simulink model "PLANT_LAB4"  (R2025b)
settings: Solver=VariableStepAuto  StartTime=0.0  StopTime=10.0  RelTol=1e-3
values from neighbouring files (symbols this model uses):
  C12 = -(batt.m*46.05+2*mot.rot.m*-7)*r    [CM_LAB4.m]
  F = [F11 F12; F12 F22]    [CM_LAB4.m]
  G2 = -(batt.m*46.05+2*mot.rot.m*-7)*g    [CM_LAB4.m]
  M11 = 2*wheel.Iyy + 2*gbox.N^2*mot.rot.Iyy+(batt.m+2*wheel.m+2*mot.m)*r^2    [CM_LAB4.m]
  M21_1 = 2*gbox.N*(1-gbox.N)*mot.rot.Iyy    [CM_LAB4.m]
  M21_2 = (batt.m*46.05+2*mot.rot.m*-7)*r    [CM_LAB4.m]
  M22 = batt.Iyy+2*(1-gbox.N)^2*mot.rot.Iyy+batt.m*46.05^2+2*mot.rot.m*49    [CM_LAB4.m]
  r = sqrt((2.20*2)/1.06)    [CM_LAB4.m]
undefined symbols (not defined in the file or in its folder): drv, g, gbox, mot, ms22g, sens, Ts
settings Model: Creator=Gioele  LastModifiedBy=Gioele

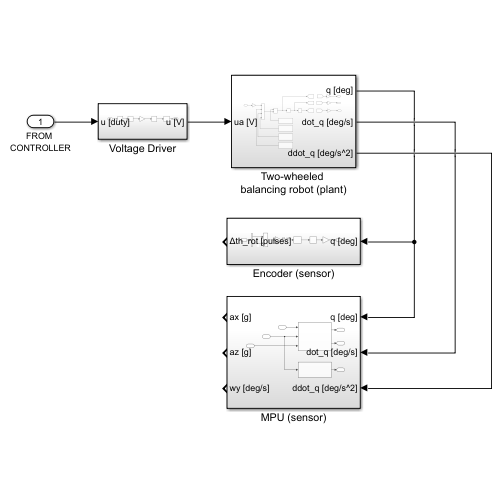
[thumbnail: Simulink's stored preview of the top-level diagram]
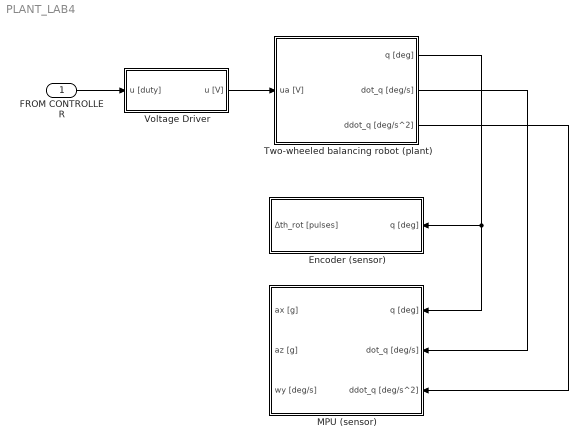
== system PLANT_LAB4 ==
  FROM CONTROLLER : Inport
  Encoder (sensor) : Subsystem
  MPU (sensor) : Subsystem
  Two-wheeled balancing robot (plant) : Subsystem
  Voltage Driver : Subsystem
  wires:
  Voltage Driver/1(u [V]) -> Two-wheeled balancing robot (plant)/1(ua [V])
  Two-wheeled balancing robot (plant)/3(ddot_q [deg/s^2]) -> MPU (sensor)/3(ddot_q [deg/s^2])
  Two-wheeled balancing robot (plant)/2(dot_q [deg/s]) -> MPU (sensor)/2(dot_q [deg/s])
  Two-wheeled balancing robot (plant)/1(q [deg]) -> MPU (sensor)/1(q [deg]), Encoder (sensor)/1(q [deg])
  FROM CONTROLLER/1 -> Voltage Driver/1(u [duty])

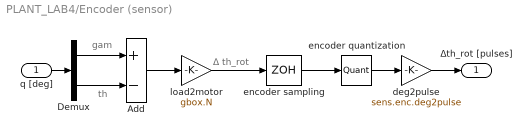
== system PLANT_LAB4/Encoder (sensor) ==
  note: Δ th_rot
  note: th
  note: gam
  q [deg] : Inport
  Add : Sum  Inputs=+-
  Demux : Demux  Outputs=2
  deg2pulse : Gain  Gain=sens.enc.deg2pulse
  encoder quantization : Quantizer  QuantizationInterval=sens.enc.pulse2deg
  encoder sampling : ZeroOrderHold  SampleTime=Ts
  load2motor : Gain  Gain=gbox.N
  Δth_rot [pulses] : Outport
  wires:
  encoder quantization/1 -> deg2pulse/1
  encoder sampling/1 -> encoder quantization/1
  load2motor/1 -> encoder sampling/1
  Demux/2 -> Add/2
  deg2pulse/1 -> Δth_rot [pulses]/1
  Demux/1 -> Add/1
  q [deg]/1 -> Demux/1
  Add/1 -> load2motor/1

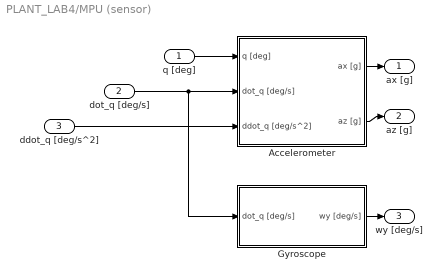
== system PLANT_LAB4/MPU (sensor) ==
  q [deg] : Inport
  dot_q [deg/s] : Inport  Port=2
  ddot_q [deg/s^2] : Inport  Port=3
  Accelerometer : Subsystem
  Gyroscope : Subsystem
  ax [g] : Outport
  az [g] : Outport  Port=2
  wy [deg/s] : Outport  Port=3
  wires:
  dot_q [deg/s]/1 -> Gyroscope/1(dot_q [deg/s]), Accelerometer/2(dot_q [deg/s])
  ddot_q [deg/s^2]/1 -> Accelerometer/3(ddot_q [deg/s^2])
  q [deg]/1 -> Accelerometer/1(q [deg])
  Gyroscope/1(wy [deg/s]) -> wy [deg/s]/1
  Accelerometer/2(az [g]) -> az [g]/1
  Accelerometer/1(ax [g]) -> ax [g]/1

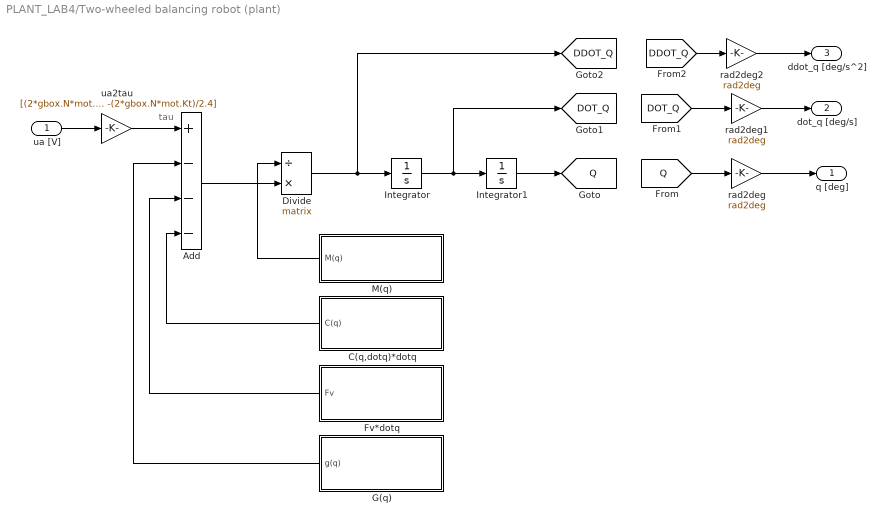
== system PLANT_LAB4/Two-wheeled balancing robot (plant) ==
  note: tau
  ua [V] : Inport
  Add : Sum  Inputs=+---
  C(q,dotq)*dotq : Subsystem
  Divide : Product  Inputs=/*  Multiplication=Matrix(*)
  Fv*dotq : Subsystem
  G(q) : Subsystem
  Integrator : Integrator
  Integrator1 : Integrator
  M(q) : Subsystem
  rad2deg : Gain  Gain=rad2deg
  rad2deg1 : Gain  Gain=rad2deg
  rad2deg2 : Gain  Gain=rad2deg
  ua2tau : Gain  Gain=[(2*gbox.N*mot.Kt)/2.4 , -(2*gbox.N*mot.Kt)/2.4]
  q [deg] : Outport
  dot_q [deg/s] : Outport  Port=2
  ddot_q [deg/s^2] : Outport  Port=3
  tag scope: DDOT_Q=global, DOT_Q=global, Q=global
  wires:
  ua2tau/1 -> Add/1
  Divide/1 -> [DDOT_Q], Integrator/1
  ua [V]/1 -> ua2tau/1
  [DOT_Q] -> rad2deg1/1
  Integrator/1 -> [DOT_Q], Integrator1/1
  Add/1 -> Divide/2
  Integrator1/1 -> [Q]
  rad2deg/1 -> q [deg]/1
  [Q] -> rad2deg/1
  [DDOT_Q] -> rad2deg2/1
  rad2deg2/1 -> ddot_q [deg/s^2]/1
  M(q)/1(M(q)) -> Divide/1
  rad2deg1/1 -> dot_q [deg/s]/1
  Fv*dotq/1(Fv) -> Add/3
  G(q)/1(g(q)) -> Add/2
  C(q,dotq)*dotq/1(C(q)) -> Add/4

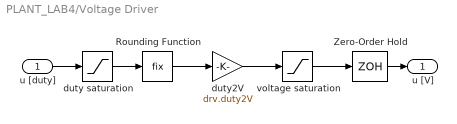
== system PLANT_LAB4/Voltage Driver ==
  u [duty] : Inport
  Rounding Function : Rounding  Operator=fix
  Zero-Order Hold : ZeroOrderHold  SampleTime=Ts
  duty saturation : Saturate  UpperLimit=drv.dutymax  LowerLimit=-drv.dutymax
  duty2V : Gain  Gain=drv.duty2V
  voltage saturation : Saturate  UpperLimit=drv.Vbus  LowerLimit=-drv.Vbus
  u [V] : Outport
  wires:
  Rounding Function/1 -> duty2V/1
  duty2V/1 -> voltage saturation/1
  duty saturation/1 -> Rounding Function/1
  Zero-Order Hold/1 -> u [V]/1
  voltage saturation/1 -> Zero-Order Hold/1
  u [duty]/1 -> duty saturation/1

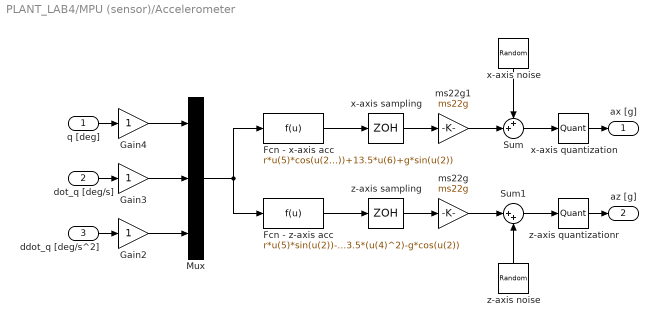
== system PLANT_LAB4/MPU (sensor)/Accelerometer ==
  q [deg] : Inport
  dot_q [deg/s] : Inport  Port=2
  ddot_q [deg/s^2] : Inport  Port=3
  Fcn - x-axis acc : Fcn  Expr=r*u(5)*cos(u(2))+13.5*u(6)+g*sin(u(2))
  Fcn - z-axis acc : Fcn  Expr=r*u(5)*sin(u(2))-13.5*(u(4)^2)-g*cos(u(2))
  Gain2 : Gain
  Gain3 : Gain
  Gain4 : Gain
  Mux : Mux  Inputs=3
  Sum : Sum  Inputs=++|
  Sum1 : Sum  Inputs=|++
  ms22g : Gain  Gain=ms22g
  ms22g1 : Gain  Gain=ms22g
  x-axis quantization : Quantizer  QuantizationInterval=sens.mpu.acc.LSB2g
  x-axis sampling : ZeroOrderHold  SampleTime=Ts
  x-axis noise : RandomNumber  Variance=sens.mpu.acc.noisevar  SampleTime=Ts
  z-axis sampling : ZeroOrderHold  SampleTime=Ts
  z-axis quantizationr : Quantizer  QuantizationInterval=sens.mpu.acc.LSB2g
  z-axis noise : RandomNumber  Variance=sens.mpu.acc.noisevar  SampleTime=Ts
  ax [g] : Outport
  az [g] : Outport  Port=2
  wires:
  x-axis noise/1 -> Sum/1
  Sum1/1 -> z-axis quantizationr/1
  x-axis sampling/1 -> ms22g1/1
  Mux/1 -> Fcn - z-axis acc/1, Fcn - x-axis acc/1
  Gain2/1 -> Mux/3
  Sum/1 -> x-axis quantization/1
  x-axis quantization/1 -> ax [g]/1
  z-axis sampling/1 -> ms22g/1
  ms22g1/1 -> Sum/2
  Gain4/1 -> Mux/1
  z-axis noise/1 -> Sum1/2
  ms22g/1 -> Sum1/1
  Fcn - x-axis acc/1 -> x-axis sampling/1
  Fcn - z-axis acc/1 -> z-axis sampling/1
  Gain3/1 -> Mux/2
  dot_q [deg/s]/1 -> Gain3/1
  z-axis quantizationr/1 -> az [g]/1
  ddot_q [deg/s^2]/1 -> Gain2/1
  q [deg]/1 -> Gain4/1

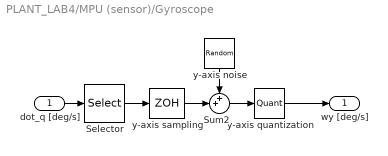
== system PLANT_LAB4/MPU (sensor)/Gyroscope ==
  dot_q [deg/s] : Inport
  Selector : Selector  InputPortWidth=2  IndexOptions=Index vector (dialog)  Indices=[2]  OutputSizes=1
  Sum2 : Sum  Inputs=++|
  y-axis quantization : Quantizer  QuantizationInterval=sens.mpu.gyro.LSB2degs
  y-axis sampling : ZeroOrderHold  SampleTime=Ts
  y-axis noise : RandomNumber  Variance=sens.mpu.gyro.noisevar  SampleTime=Ts
  wy [deg/s] : Outport
  wires:
  Selector/1 -> y-axis sampling/1
  y-axis noise/1 -> Sum2/1
  dot_q [deg/s]/1 -> Selector/1
  Sum2/1 -> y-axis quantization/1
  y-axis sampling/1 -> Sum2/2
  y-axis quantization/1 -> wy [deg/s]/1

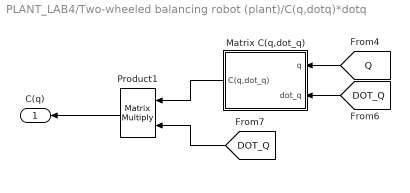
== system PLANT_LAB4/Two-wheeled balancing robot (plant)/C(q,dotq)*dotq ==
  Matrix C(q,dot_q) : Subsystem
  Product1 : Product  Multiplication=Matrix(*)
  C(q) : Outport
  wires:
  [Q] -> Matrix C(q,dot_q)/1(q)
  Matrix C(q,dot_q)/1(C(q,dot_q)) -> Product1/1
  [DOT_Q] -> Product1/2
  Product1/1 -> C(q)/1
  [DOT_Q] -> Matrix C(q,dot_q)/2(dot_q)

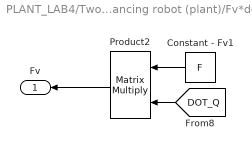
== system PLANT_LAB4/Two-wheeled balancing robot (plant)/Fv*dotq ==
  Constant - Fv1 : Constant  Value=F
  Product2 : Product  Multiplication=Matrix(*)
  Fv : Outport
  wires:
  Constant - Fv1/1 -> Product2/1
  [DOT_Q] -> Product2/2
  Product2/1 -> Fv/1

== system PLANT_LAB4/Two-wheeled balancing robot (plant)/G(q) ==
  Matrix g(q) : Subsystem
  g(q) : Outport
  wires:
  [Q] -> Matrix g(q)/1(q)
  Matrix g(q)/1(g(q)) -> g(q)/1

== system PLANT_LAB4/Two-wheeled balancing robot (plant)/M(q) ==
  Matrix M(q) : Subsystem
  M(q) : Outport
  wires:
  [Q] -> Matrix M(q)/1(q)
  Matrix M(q)/1(M(q)) -> M(q)/1

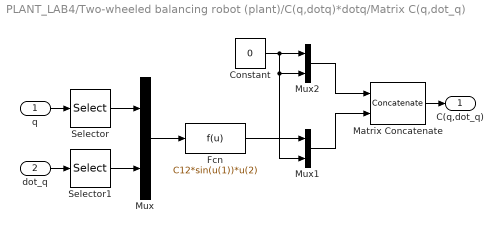
== system PLANT_LAB4/Two-wheeled balancing robot (plant)/C(q,dotq)*dotq/Matrix C(q,dot_q) ==
  q : Inport
  dot_q : Inport  Port=2
  Constant : Constant  Value=0
  Fcn : Fcn  Expr=C12*sin(u(1))*u(2)
  Matrix Concatenate : Concatenate  Mode=Multidimensional array  ConcatenateDimension=2
  Mux : Mux  Inputs=2
  Mux1 : Mux  Inputs=2
  Mux2 : Mux  Inputs=2
  Selector : Selector  InputPortWidth=2  IndexOptions=Index vector (dialog)  Indices=[2]  OutputSizes=1
  Selector1 : Selector  InputPortWidth=2  IndexOptions=Index vector (dialog)  Indices=[2]  OutputSizes=1
  C(q,dot_q) : Outport
  wires:
  Selector1/1 -> Mux/2
  Mux/1 -> Fcn/1
  Constant/1 -> Mux2/2, Mux1/2, Mux2/1
  Mux2/1 -> Matrix Concatenate/1
  Selector/1 -> Mux/1
  Mux1/1 -> Matrix Concatenate/2
  Fcn/1 -> Mux1/1
  Matrix Concatenate/1 -> C(q,dot_q)/1
  dot_q/1 -> Selector1/1
  q/1 -> Selector/1

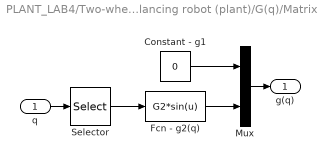
== system PLANT_LAB4/Two-wheeled balancing robot (plant)/G(q)/Matrix g(q) ==
  q : Inport
  Constant - g1 : Constant  Value=0
  Fcn - g2(q) : Fcn  Expr=G2*sin(u)
  Mux : Mux  Inputs=2
  Selector : Selector  InputPortWidth=2  IndexOptions=Index vector (dialog)  Indices=[2]  OutputSizes=1
  g(q) : Outport
  wires:
  Selector/1 -> Fcn - g2(q)/1
  Constant - g1/1 -> Mux/1
  Mux/1 -> g(q)/1
  Fcn - g2(q)/1 -> Mux/2
  q/1 -> Selector/1

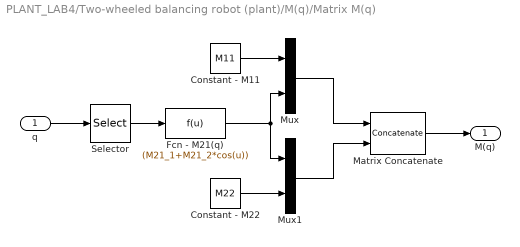
== system PLANT_LAB4/Two-wheeled balancing robot (plant)/M(q)/Matrix M(q) ==
  q : Inport
  Constant - M11 : Constant  Value=M11
  Constant - M22 : Constant  Value=M22
  Fcn - M21(q) : Fcn  Expr=(M21_1+M21_2*cos(u))
  Matrix Concatenate : Concatenate  Mode=Multidimensional array  ConcatenateDimension=2
  Mux : Mux  Inputs=2
  Mux1 : Mux  Inputs=2
  Selector : Selector  InputPortWidth=2  IndexOptions=Index vector (dialog)  Indices=[2]  OutputSizes=1
  M(q) : Outport
  wires:
  Matrix Concatenate/1 -> M(q)/1
  Selector/1 -> Fcn - M21(q)/1
  Fcn - M21(q)/1 -> Mux/2, Mux1/1
  Constant - M11/1 -> Mux/1
  q/1 -> Selector/1
  Constant - M22/1 -> Mux1/2
  Mux1/1 -> Matrix Concatenate/2
  Mux/1 -> Matrix Concatenate/1
